simulink model "TX_ESP32"  (R2025b)
settings: Solver=FixedStepDiscrete  StartTime=0.0  StopTime=30  FixedStep=0.1  RelTol=1e-3
libraries: instrumentseriallib x2, svdutilitieslib x1
settings Model: Creator=daniel.camacho  LastModifiedBy=daniel.camacho

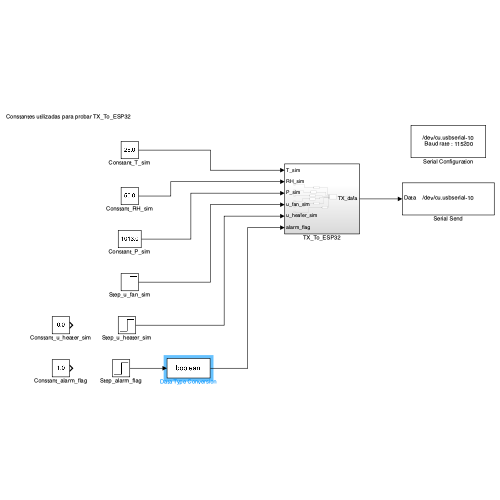
[thumbnail: Simulink's stored preview of the top-level diagram]
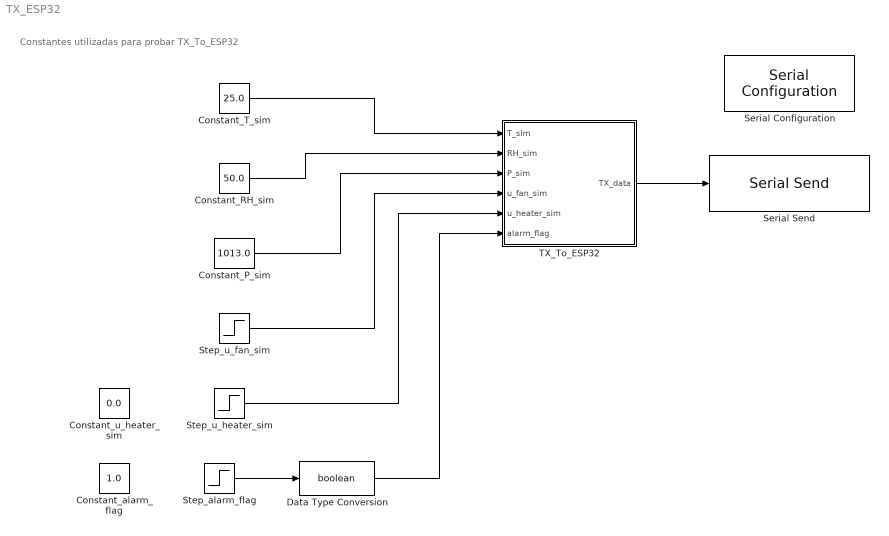
== system TX_ESP32 ==
  note: Constantes utilizadas para probar TX_To_ESP32
  Constant_P_sim : Constant  Value=1013.0  OutDataTypeStr=double
  Constant_RH_sim : Constant  Value=50.0  OutDataTypeStr=double
  Constant_T_sim : Constant  Value=25.0  OutDataTypeStr=double
  Constant_alarm_flag : Constant  Value=1.0  OutDataTypeStr=boolean
  Constant_u_heater_sim : Constant  Value=0.0  OutDataTypeStr=double
  Data Type Conversion : DataTypeConversion  OutDataTypeStr=boolean  SaturateOnIntegerOverflow=off  RndMeth=Floor
  Serial Configuration : instrumentseriallib/Serial Configuration  Priority=-200000  PortSel=/dev/cu.usbserial-10  Port=/dev/cu.usbserial-10  ComPort=/dev/cu.usbserial-10  BaudRate=115200  DataBits=8  Parity=none  StopBits=1  ByteOrder=little-endian  FlowControl=none  Timeout=10  SimulateUsing=Interpreted execution  BlockInModel=on  aMode=1
  Serial Send : instrumentseriallib/Serial Send  Priority=1  PortSel=/dev/cu.usbserial-10  Port=/dev/cu.usbserial-10  ComPort=/dev/cu.usbserial-10  Header=[]  Terminator=<none>  CustomTerminator=[]  EnableBlockingMode=on  SimulateUsing=Interpreted execution  BlockInModel=on  aMode=1
  Step_alarm_flag : Step  Time=15  OutDataTypeStr=single  SampleTime=0.1
  Step_u_fan_sim : Step  Time=10  After=0.8  SampleTime=0.1
  Step_u_heater_sim : Step  Time=10  After=0.8  SampleTime=0.1
  TX_To_ESP32 : Subsystem
  wires:
  Step_u_fan_sim/1 -> TX_To_ESP32/4(u_fan_sim)
  Constant_RH_sim/1 -> TX_To_ESP32/2(RH_sim)
  Constant_T_sim/1 -> TX_To_ESP32/1(T_sim)
  Constant_P_sim/1 -> TX_To_ESP32/3(P_sim)
  TX_To_ESP32/1(TX_data) -> Serial Send/1
  Step_u_heater_sim/1 -> TX_To_ESP32/5(u_heater_sim)
  Step_alarm_flag/1 -> Data Type Conversion/1
  Data Type Conversion/1 -> TX_To_ESP32/6(alarm_flag)

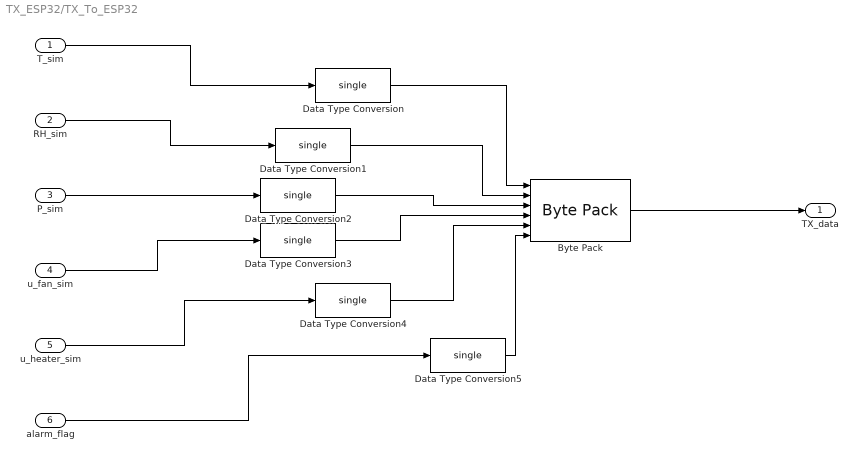
== system TX_ESP32/TX_To_ESP32 ==
  T_sim : Inport  OutDataTypeStr=double
  RH_sim : Inport  Port=2  OutDataTypeStr=double
  P_sim : Inport  Port=3  OutDataTypeStr=double
  u_fan_sim : Inport  Port=4  OutDataTypeStr=double
  u_heater_sim : Inport  Port=5  OutDataTypeStr=double
  alarm_flag : Inport  Port=6  OutDataTypeStr=boolean
  Byte Pack : svdutilitieslib/Byte Pack  maskPackedDataType=uint8  datatypes={'single', 'single', 'single', 'single', 'single', 'single'}  byteAlign=1  blockPlatform=arduinoert
  Data Type Conversion{,1..5} (6 alike) : DataTypeConversion  OutDataTypeStr=single  SaturateOnIntegerOverflow=off  RndMeth=Floor
  TX_data : Outport  OutDataTypeStr=uint8
  wires:
  T_sim/1 -> Data Type Conversion/1
  RH_sim/1 -> Data Type Conversion1/1
  P_sim/1 -> Data Type Conversion2/1
  u_fan_sim/1 -> Data Type Conversion3/1
  u_heater_sim/1 -> Data Type Conversion4/1
  alarm_flag/1 -> Data Type Conversion5/1
  Byte Pack/1 -> TX_data/1
  Data Type Conversion/1 -> Byte Pack/1
  Data Type Conversion1/1 -> Byte Pack/2
  Data Type Conversion2/1 -> Byte Pack/3
  Data Type Conversion3/1 -> Byte Pack/4
  Data Type Conversion4/1 -> Byte Pack/5
  Data Type Conversion5/1 -> Byte Pack/6
